simulink model "Revised_EGPPROPOSEDMODEL"  (R2022a)
settings: Solver=VariableStepAuto  StartTime=0.0  StopTime=24*60  RelTol=1e-3
values from neighbouring files (symbols this model uses):
  AG = 0.8    [RevisedEGPproposed.m]
  G10 = 90    [RevisedEGPproposed.m]
  Gb = 90    [RevisedEGPproposed.m]
  Ggnb = .495    (= 0.495)    [RevisedEGPproposed.m]
  Hb = 5.8/(10^6)    (= 5.8e-06)    [RevisedEGPproposed.m]
  I0 = (u0)/(70*.01656)    (= 11.1393202208)    [RevisedEGPproposed.m]
  K12 = 0.066    [RevisedEGPproposed.m]
  K6GP = 0.034    [RevisedEGPproposed.m]
  KA1 = 0.006    [RevisedEGPproposed.m]
  KA2 = 0.06    [RevisedEGPproposed.m]
  KA3 = 0.03    [RevisedEGPproposed.m]
  KB1 = KA1*S1T    (= 3.072e-05)    [RevisedEGPproposed.m]
  KB2 = KA2*S1D    (= 4.92e-05)    [RevisedEGPproposed.m]
  KB3 = SIE*KA3    (= 0.00156)    [RevisedEGPproposed.m]
  Ke = 0.138    [RevisedEGPproposed.m]
  s10 = u0*TmaxI    (= 710.1985)    [RevisedEGPproposed.m]
  s20 = s10    (= 710.1985)    [RevisedEGPproposed.m]
  tD = 40    [RevisedEGPproposed.m]
  TmaxI = 55    [RevisedEGPproposed.m]
  VG = 0.16*70    (= 11.2)    [RevisedEGPproposed.m]
  VI = 0.12*70    (= 8.4)    [RevisedEGPproposed.m]
  x10 = (.30898*u0)/70    (= 0.0569966578)    [RevisedEGPproposed.m]
  x20 = (.04951*u0)/70    (= 0.00913296824286)    [RevisedEGPproposed.m]
  x30 = (3.2206*u0)/70    (= 0.594094880286)    [RevisedEGPproposed.m]
settings Model: Creator=Artificial_Pancreas  LastModifiedBy=Acer
settings ModelReferenceCC: EnableRefExpFcnMdlSchedulingChecks=off
settings RTWCC: Description=Generic Real-Time Target

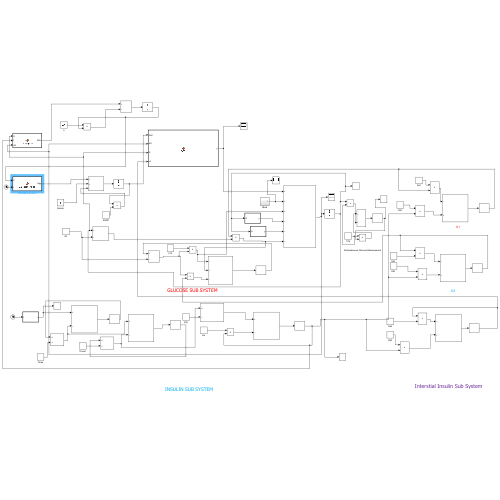
[thumbnail: Simulink's stored preview of the top-level diagram]
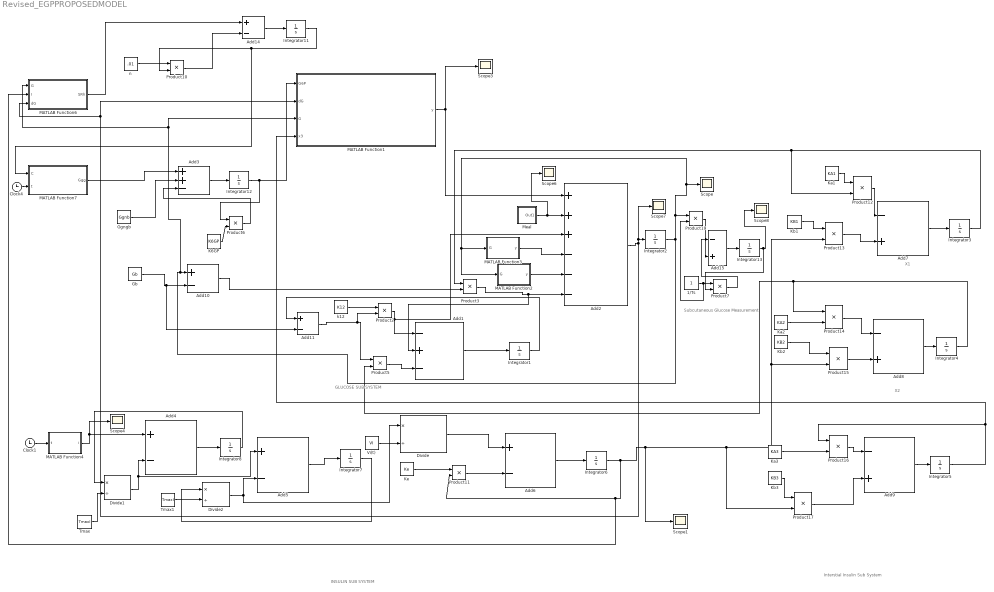
== system Revised_EGPPROPOSEDMODEL ==
  note: Subcutaneous Glucose Measurement
  note: X2
  note: X1
  note: Interstial Insulin Sub System
  note: INSULIN SUB SYSTEM
  note: GLUCOSE SUB SYSTEM
  1/Ts : Constant
  Add1 : Sum  Inputs=-+-
  Add{4..6,10..11,14} (6 alike) : Sum  Inputs=+-
  Add{7..9,15} (4 alike) : Sum  Inputs=-+
  Add2 : Sum  Inputs=+++---
  Add3 : Sum  Inputs=++-
  Clock1 : Clock
  Clock4 : Clock
  Divide : Product  Inputs=*/  RndMeth=Zero  SaturateOnIntegerOverflow=on
  Divide1 : Product  Inputs=*/  RndMeth=Zero  SaturateOnIntegerOverflow=on
  Divide2 : Product  Inputs=*/  RndMeth=Zero  SaturateOnIntegerOverflow=on
  Gb : Constant  Value=Gb
  Ggngb : Constant  Value=Ggnb
  Integrator1 : Integrator  InitialCondition=70
  Integrator11 : Integrator  InitialCondition=Hb
  Integrator12 : Integrator  InitialCondition=41.897
  Integrator13 : Integrator  InitialCondition=Gb
  Integrator2 : Integrator  InitialCondition=G10
  Integrator3 : Integrator  InitialCondition=x10
  Integrator4 : Integrator  InitialCondition=x20
  Integrator5 : Integrator  InitialCondition=x30
  Integrator6 : Integrator  InitialCondition=I0
  Integrator7 : Integrator  InitialCondition=s20
  Integrator8 : Integrator  InitialCondition=s10
  K6GP : Constant  Value=K6GP
  Ka1 : Constant  Value=KA1
  Ka2 : Constant  Value=KA2
  Ka3 : Constant  Value=KA3
  Kb1 : Constant  Value=KB1
  Kb2 : Constant  Value=KB2
  Kb3 : Constant  Value=KB3
  Ke : Constant  Value=Ke
  MATLAB Function1 : MATLAB Function  TreatAsAtomicUnit=on
  MATLAB Function2 : MATLAB Function  TreatAsAtomicUnit=on
  MATLAB Function3 : MATLAB Function  TreatAsAtomicUnit=on
  MATLAB Function4 : MATLAB Function  TreatAsAtomicUnit=on
  MATLAB Function6 : MATLAB Function  TreatAsAtomicUnit=on
  MATLAB Function7 : MATLAB Function  TreatAsAtomicUnit=on
  Meal : Subsystem
  Product{2..3,5..7,10..17,19} (14 alike) : Product
  Scope{,1,3..4,6..8} (7 alike) : Scope
  Tmax : Constant  Value=TmaxI
  Tmax1 : Constant  Value=TmaxI
  Vi(t) : Constant  Value=VI
  k12 : Constant  Value=K12
  n : Constant  Value=.01
  wires:
  Product5/1 -> Add1/3
  Product2/1 -> Add2/3, Add1/1
  Add2/1 -> Integrator2/1, Scope7/1, MATLAB Function1/2(dG), MATLAB Function6/3(dG)
  Vi(t)/1 -> Divide/2
  Divide/1 -> Add6/1
  Product11/1 -> Add6/2
  Ke/1 -> Product11/1
  Product12/1 -> Add7/1
  Product13/1 -> Add7/2
  Kb1/1 -> Product13/1
  Ka1/1 -> Product12/1
  Kb2/1 -> Product15/1
  Product15/1 -> Add8/2
  Product14/1 -> Add8/1
  Kb3/1 -> Product17/1
  Product17/1 -> Add9/2
  Product16/1 -> Add9/1
  Add7/1 -> Integrator3/1
  Add8/1 -> Integrator4/1
  Ka3/1 -> Product16/2
  Add9/1 -> Integrator5/1
  Add6/1 -> Integrator6/1
  Integrator6/1 -> MATLAB Function6/2(I), Product11/2, Scope1/1, Product17/2, Product15/2, Product13/2
  Add4/1 -> Integrator8/1
  Integrator8/1 -> Divide1/1
  Add5/1 -> Integrator7/1
  Divide1/1 -> Add4/2, Add5/1
  Divide2/1 -> Add5/2, Divide/1
  Tmax/1 -> Divide1/2
  Tmax1/1 -> Divide2/2
  Integrator7/1 -> Divide2/1
  k12/1 -> Product2/1
  Integrator3/1 -> Product12/2, Product3/1
  Integrator4/1 -> Product14/1, Product5/2
  Integrator5/1 -> MATLAB Function1/4(x3), Product16/1
  Integrator2/1 -> MATLAB Function6/1(G), MATLAB Function1/3(G), Add10/1, Product19/1, MATLAB Function2/1(G), MATLAB Function3/1(G), Scope/1
  Add1/1 -> Integrator1/1
  Integrator1/1 -> Add11/1
  MATLAB Function2/1(y) -> Add2/5
  Product3/1 -> Add1/2, Add2/6
  Add10/1 -> Product3/2
  Gb/1 -> Add11/2, Add10/2
  Add11/1 -> Product5/1, Product2/2
  Ka2/1 -> Product14/2
  Clock1/1 -> MATLAB Function4/1(t)
  MATLAB Function4/1(i) -> Add4/1, Scope4/1
  MATLAB Function3/1(y) -> Add2/4
  MATLAB Function1/1(y) -> Add2/1, Scope3/1
  n/1 -> Product10/1
  Add14/1 -> Integrator11/1
  Product10/1 -> Add14/2
  MATLAB Function6/1(SRh) -> Add14/1
  Integrator11/1 -> MATLAB Function7/1(C), Product10/2
  Clock4/1 -> MATLAB Function7/2(t)
  MATLAB Function7/1(Ggg) -> Add3/1
  Ggngb/1 -> Add3/2
  Add3/1 -> Integrator12/1
  Integrator12/1 -> MATLAB Function1/1(G6P), Product6/1
  K6GP/1 -> Product6/2
  Product6/1 -> Add3/3
  Add15/1 -> Integrator13/1
  Integrator13/1 -> Product7/2, Scope8/1
  1/Ts/1 -> Product19/2, Product7/1
  Product7/1 -> Add15/1
  Product19/1 -> Add15/2
  Meal/1(Out1) -> Scope6/1, Add2/2

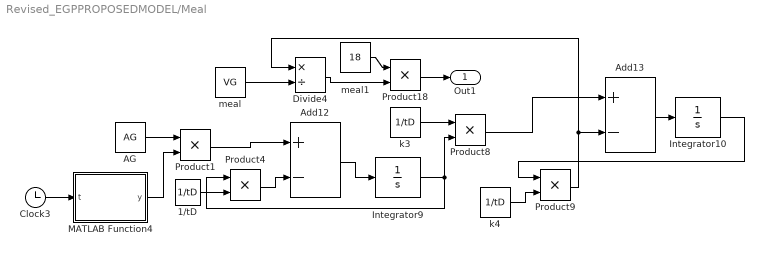
== system Revised_EGPPROPOSEDMODEL/Meal ==
  1/tD : Constant  Value=1/tD
  AG : Constant  Value=AG
  Add12 : Sum  Inputs=+-
  Add13 : Sum  Inputs=+-
  Clock3 : Clock
  Divide4 : Product  Inputs=*/  RndMeth=Zero  SaturateOnIntegerOverflow=on
  Integrator10 : Integrator
  Integrator9 : Integrator
  MATLAB Function4 : MATLAB Function  TreatAsAtomicUnit=on
  Product{1,4,8..9,18} (5 alike) : Product
  k3 : Constant  Value=1/tD
  k4 : Constant  Value=1/tD
  meal : Constant  Value=VG
  meal1 : Constant  Value=18
  Out1 : Outport
  wires:
  AG/1 -> Product1/1
  meal1/1 -> Product18/1
  meal/1 -> Divide4/2
  Product1/1 -> Add12/1
  1/tD/1 -> Product4/2
  MATLAB Function4/1(y) -> Product1/2
  k3/1 -> Product8/1
  Divide4/1 -> Product18/2
  k4/1 -> Product9/2
  Product9/1 -> Divide4/1, Add13/2
  Integrator9/1 -> Product4/1, Product8/2
  Clock3/1 -> MATLAB Function4/1(t)
  Product18/1 -> Out1/1
  Product4/1 -> Add12/2
  Add13/1 -> Integrator10/1
  Integrator10/1 -> Product9/1
  Product8/1 -> Add13/1
  Add12/1 -> Integrator9/1

== matlab function Revised_EGPPROPOSEDMODEL/MATLAB Function1 ==
  data: y output; G6P input; dG input; G input; x3 input
function y = EGP(G6P,dG,G,x3)
% Parameter values

Gb=90;                %mg/dL
% Ggnb = .495 ;        %mg/dL/min
Gggb =    0.7425;     %mg/dL/min
Sc = 306;        %mg/dl/mim per mg/dl
Cth = 80*10^-7       %mg/dL        
K6GP = 0.034         %/min
tD = 59.90          % min
tau = 23.24          % min
kp2 = 0.0007;                %mg/dL
%  if G <= Gb
%     E = 1/2 *(1-tanh((t-tD)/tau));
%     
%     Ggg = Gggb + (Sc * max(0, (C - Cth)).*E)
%     
if dG>=0
     y = K6GP*G6P -kp2*(G -Gb)-x3.*dG;
 %  y = K6GP*G6P
%   y = Ggnb + Ggg- x3.*dG -kp2*(G -Gb)-x3.*(G -Gb);
% y = Ggnb + x3.*Ggg- x3.*dG -kp2*(G -Gb);
  else
        y = K6GP*G6P -kp2*(G -Gb);
%         y = Ggnb + Ggg -kp2*(G -Gb)-x3.*(G -Gb);
%     y = Ggnb + x3.*Ggg -kp2*(G -Gb);
%     end
%     else 
%         if dG>=0
% %     y = Ggnb + Ggg- x3.*dG -kp2*(G -Gb)-x3.*(G -Gb);
% y = Ggnb - x3.*dG -kp2*(G -Gb);
%     else
% %         y = Ggnb + Ggg -kp2*(G -Gb)-x3.*(G -Gb);
%     y = Ggnb-kp2*(G -Gb);
    
            end

== matlab function Revised_EGPPROPOSEDMODEL/MATLAB Function6 ==
  data: SRh output; G input; I input; dG input
function SRh  = GlucagonS(G,I,dG)
 Gb=90;              %mg/dL
Gth=60;             %mg/dL
n=0.01;              %per minute
Hb=5.8/(10^6);       %mg/dL
P=0.86;              %per minute  
VI = 0.12*70;
sigma= 1/(10^9*6.945*VI);     %mg/dL/min
delta=0.98;              %mg/dL
Srhbd=0;
G=Gb;                %mg/dL
H=Hb;
SRhb=n*Hb;
SRhs=SRhb;

%Equations
% for t=1:1000
    
    if G>=Gb
        SRhs=P*(SRhs-SRhb);
    
    else
        SRhs=P*(SRhs-max(((sigma*(Gth-G)/(I+1))+SRhb),0));
    end

    SRhd=delta*max (-dG,0);

    SRh=SRhs+SRhd;
   
end

== matlab function Revised_EGPPROPOSEDMODEL/MATLAB Function2 ==
  data: y output; G input
function y = kidney(G)
Ke1=0.003; Ke2=162; 
% VG = 0.16;
if (G>=Ke2)
     y=Ke1.*(G-Ke2);
else
         y=0;
         
end
end

== matlab function Revised_EGPPROPOSEDMODEL/MATLAB Function3 ==
  data: y output; G input
function y = Insulinindependent(G)
 F01 =18*((.00097*70)/(0.12*70));
if (G>=81)
        y=F01;
else
         y= (F01).*(G/81);

end

== matlab function Revised_EGPPROPOSEDMODEL/MATLAB Function4 ==
  data: t input; i output
function i = insulin(t)
 if t<210
    i=12.9127;
  elseif   (t>=210) && (t<=215)
   i=700;
%    elseif   (t>=390) && (t<=395)
elseif   (t>=450) && (t<=455)
   i=250;
%    elseif   (t>=600) && (t<=605)
 elseif   (t>=690) && (t<=695)
   i=200;
%    elseif   (t>=765) && (t<=770)
%    i=490;
%    elseif   (t>=900) && (t<=905)
%    i=210;
 else i= 12.9127;

%% formula used to calculate insulin
 % body_weight =70;
% TDD = 0.55*body_weight;
% ICR = 500/TDD;
% % ICR = 500/TDD;
% ISF = 1800/TDD;
% Breakfast_m1 = 30;
% Lunch_m2 = 60;
% Dinner_m3 = 40;
% m1_bolus = Breakfast_m1 / ICR;
% m2_bolus = Lunch_m2/ICR;
% m3_bolus = Dinner_m3/ICR;
% Average_m = (m1_bolus+m2_bolus+m3_bolus)/3;
% Active_insulin = (Average_m)/body_weight;
% %  Active_insulin = 6/body_weight;

% BG_target1 = 100;
% BG_current1 = 96.7;
% Correction_bolus1 = (BG_current1 - BG_target1)/ISF;
% i= ((m1_bolus +Correction_bolus1 -Active_insulin) *10^6)/10;
% i= i1/(24*60)
% i=(18.15 *10^6)/(24*60)
%   i=0.0140*10^6;
% elseif (t>=470) && (t<=480)
%     i=0;
% BG_target2 = 100;
% BG_current2 = 103;
% Correction_bolus2 = (BG_current2 - BG_target2)/ISF;
% i= ((m2_bolus +Correction_bolus2 -Active_insulin)*10^6)/10;
% % %  i=0.2098*10^6;
% elseif (t>=890) && (t<=900)
%     BG_target3 = 100;
% BG_current3 = 102;
% Correction_bolus3 = (BG_current3 - BG_target3)/ISF;
% i= ((m3_bolus +Correction_bolus3 -Active_insulin)*10^6)/10;
% % %     i=0;
% % %  i=0.0299*10^6;
% else
%    i=0;
end
end

== matlab function Revised_EGPPROPOSEDMODEL/MATLAB Function7 ==
  data: Ggg output; C input; t input
function Ggg  = GlucagenolysisS(C,t)
Gb=90;                %mg/dL
% Ggnb = .495 ;        %mg/dL/min
Gggb =    0.7425;     %mg/dL/min
Sc = 297;        %mg/dl/mim per mg/dl
Cth = 80*10^-7       %mg/dL        
K6GP = 0.034         %/min
tD = 59.90          % min
tau = 23.24         % min
kp2 = 0.0007;                %mg/dL
%  if G <= Gb
   E = 1/2 *(1-tanh((t-tD)/tau));
% E = 1;
    Ggg = [Gggb + (Sc * max(0, (C - Cth)))].*E
   
end

== matlab function Revised_EGPPROPOSEDMODEL/Meal/MATLAB Function4 ==
  data: t input; y output
function y = meal(t)
d1 = 12.42; 
Dg1=(1000*d1)/180;
d2 = 1.83; 
Dg2=(1000*d2)/180;
d3 = 3.45; 
Dg3=(1000*d3)/180;
% d4 = 3.85; 
% Dg4=(1000*d4)/180;
% d5 = 3.45; 
% Dg5=(1000*d5)/180;
if (t<210)
    y=0;
 elseif   (t>=210) && (t<220)
y=Dg1;
% elseif t>=390 && t<=410
elseif t>=450 && t<=470
        y=Dg2;
%     elseif t>=600 && t<=610
        elseif t>=690 && t<=700
       y=Dg3;
%     elseif t>=765 && t<=785
%         y=Dg4;
%     elseif t>=900 && t<=910
%        y=Dg5;
  else
    y=0;
end
